simulink subsystem "ego_vehicle_info"  (R2022b)
settings: Solver=VariableStepAuto  StartTime=0.0  StopTime=10.0  RelTol=1e-3
libraries: CarMaker4SL x4
settings Model: Creator=USER  LastModifiedBy=USER

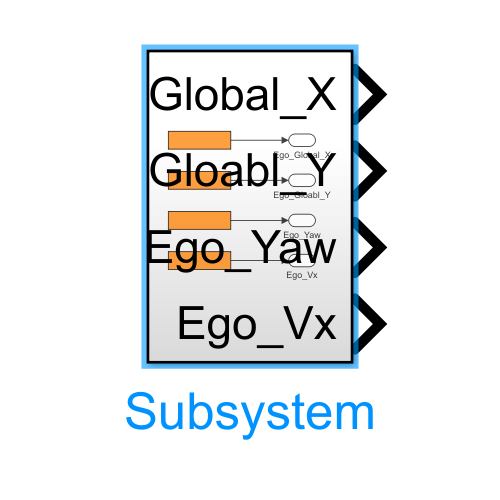
[thumbnail: Simulink's stored preview of the top-level diagram]
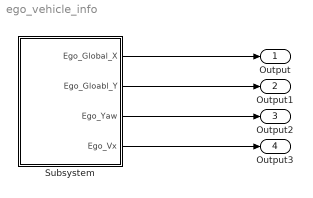
== system ego_vehicle_info ==
  Subsystem : Subsystem
  Output : Outport
  Output1 : Outport  Port=2
  Output2 : Outport  Port=3
  Output3 : Outport  Port=4
  wires:
  Subsystem/1(Ego_Global_X) -> Output/1
  Subsystem/2(Ego_Gloabl_Y) -> Output1/1
  Subsystem/3(Ego_Yaw) -> Output2/1
  Subsystem/4(Ego_Vx) -> Output3/1

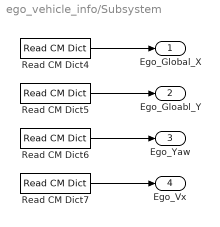
== system ego_vehicle_info/Subsystem ==
  Read CM Dict4 : CarMaker4SL/Read CM Dict  xname=Car.Fr1.tx  xsync=off  xstime=Inherited
  Read CM Dict5 : CarMaker4SL/Read CM Dict  xname=Car.Fr1.ty  xsync=off  xstime=Inherited
  Read CM Dict6 : CarMaker4SL/Read CM Dict  xname=Car.Fr1.rz  xsync=off  xstime=Inherited
  Read CM Dict7 : CarMaker4SL/Read CM Dict  xname=Car.v  xsync=off  xstime=Inherited
  Ego_Global_X : Outport
  Ego_Gloabl_Y : Outport  Port=2
  Ego_Yaw : Outport  Port=3
  Ego_Vx : Outport  Port=4
  wires:
  Read CM Dict4/1 -> Ego_Global_X/1
  Read CM Dict5/1 -> Ego_Gloabl_Y/1
  Read CM Dict6/1 -> Ego_Yaw/1
  Read CM Dict7/1 -> Ego_Vx/1
